simulink model "sim_test"  (R2023b)
settings: Solver=FixedStepAuto  StartTime=0.0  StopTime=20  FixedStep=1  RelTol=1e-3
InitFcn:
  | init
libraries: instrumentseriallib x2, SignalEditorBlockLib x1
settings Model: Creator=Elias  LastModifiedBy=Elias
settings HardwareCC: ProdBitPerLong=64  ProdHWDeviceType=Intel->x86-64 (Linux 64)
settings RTWCC: Description=Simulink Desktop Real-Time  SystemTargetFile=sldrt.tlc  TemplateMakefile=sldrt.tmf  RTWCompilerOptimization=on
settings CodeAppCC: MaxIdLength=95
settings SimulinkDesktopRealTimeCC: TargetLibSuffix=_sldrt.a  TargetPreCompLibLocation=C:\Program Files\MATLAB\R2023b\toolbox\sldrt\lib\win64

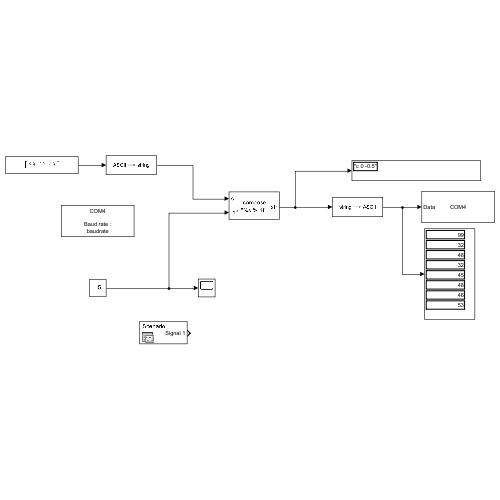
[thumbnail: Simulink's stored preview of the top-level diagram]
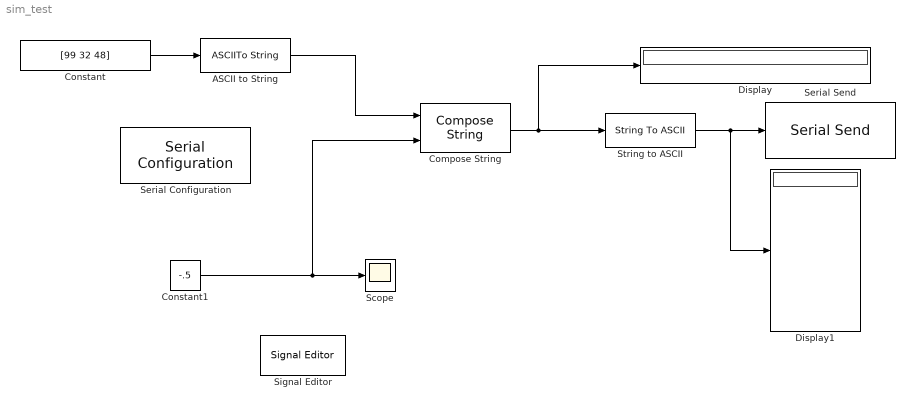
== system sim_test ==
  ASCII to String : ASCIIToString
  Compose String : ComposeString  Format="\"%s %.1f\""
  Constant : Constant  Value=[99 32 48]  VectorParams1D=off  OutDataTypeStr=uint8
  Constant1 : Constant  Value=-.5
  Display : Display
  Display1 : Display
  Scope : Scope
  Serial Configuration : instrumentseriallib/Serial Configuration  Priority=-200000  PortSel=port  Port=port  ComPort=port  BaudRate=baudrate  DataBits=8  Parity=none  StopBits=1  ByteOrder=little-endian  FlowControl=none  Timeout=2  SimulateUsing=Interpreted execution  BlockInModel=on  aMode=1
  Serial Send : instrumentseriallib/Serial Send  Priority=1  PortSel=port  Port=port  ComPort=port  Header=[]  Terminator=<none>  CustomTerminator=[]  EnableBlockingMode=on  SimulateUsing=Interpreted execution  BlockInModel=on  aMode=1
  Signal Editor : SignalEditorBlockLib/Signal Editor  FileName=noe.mat  ActiveScenario=Scenario  ActiveSignal=Signal 1  IsBus=off  OutputBusObjectStr=Bus: BusObject  SampleTime=0  ZeroCross=off  OutputAfterFinalValue=Holding final value  Unit=inherit  PreserveSignalName=on  ApplySigPropsToAllScenarios=on  ApplySigPropsToAllSignals=off
  String to ASCII : StringToASCII  OutputVectorSize=8
  wires:
  Constant1/1 -> Compose String/2, Scope/1
  Constant/1 -> ASCII to String/1
  ASCII to String/1 -> Compose String/1
  Compose String/1 -> String to ASCII/1, Display/1
  String to ASCII/1 -> Display1/1, Serial Send/1
